simulink model "builtin_block_model_Shunt"  (R2023b)
settings: Solver=VariableStepAuto  StartTime=0.0  StopTime=10  RelTol=1e-3
values from neighbouring files (symbols this model uses):
  J = 0.21    [setup_params_shunt.m]
  LAA = 0.01    [setup_params_shunt.m]
  LFF = 0.167    [setup_params_shunt.m]
  ra = 0.013    [setup_params_shunt.m]
  rf = 1.43    [setup_params_shunt.m]
  Tl = 2.493    [setup_params_shunt.m]
  Va = 24    [setup_params_shunt.m]
libraries: spsControlledVoltageSourceLib x1, spsDCMachineLib x1, sps_lib x1
settings Model: Creator=Noor  LastModifiedBy=USER
settings SolverCC: AlgebraicLoopSolver=TrustRegion
settings DataIOCC: ReturnWorkspaceOutputs=off
settings DebuggingCC: UnconnectedInputMsg=warning  UnconnectedOutputMsg=warning  UnconnectedLineMsg=warning  ArithmeticOperatorsInVariantConditions=warning
settings ModelReferenceCC: EnableRefExpFcnMdlSchedulingChecks=on
settings SFSimCC: SimUseLocalCustomCode=off  CustomCodeUndefinedFunction=UseInterfaceOnly
settings RTWCC: RTWUseLocalCustomCode=off

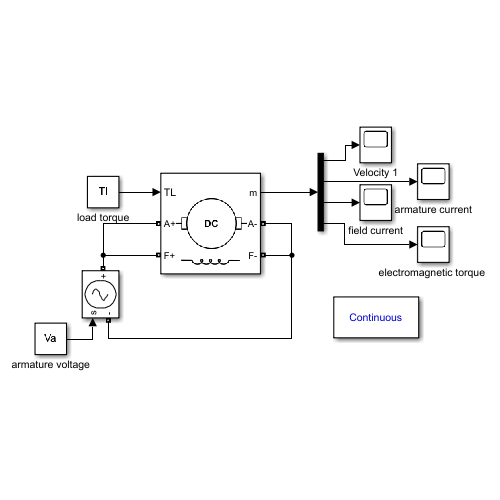
[thumbnail: Simulink's stored preview of the top-level diagram]
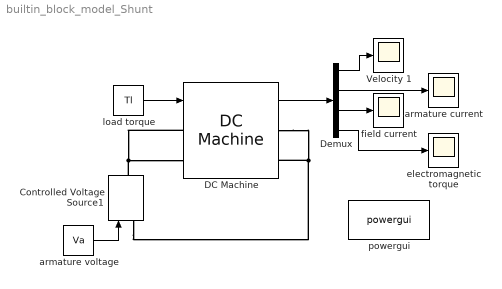
== system builtin_block_model_Shunt ==
  Controlled Voltage Source1 : spsControlledVoltageSourceLib/Controlled Voltage Source  Initialize=on  Source_Type=AC  Amplitude=0  Phase=0  Frequency=0  Measurements=None
  DC Machine : spsDCMachineLib/DC Machine  PresetModel=No  MechanicalLoad=Torque TL  FieldType=Wound  ShowDetailedParameters=on  MeasurementBus=off  RLa=[ra LAA]  RLf=[rf LFF]  Laf=LAF  MachineConstant=Torque constant (N.m/A)  Ke=1.8  Kt=1.8  J=J  Bm=Bm  Tf=0  w0=0  Ifinit=0  TsPowergui=0  TsBlock=-1
  Demux : Demux
  Velocity 1 : Scope
  armature current : Scope
  armature voltage : Constant  Value=Va
  "electromagnetic torque " : Scope
  field current : Scope
  load torque : Constant  Value=Tl
  powergui : sps_lib/powergui  Priority=1  SimulationMode=Continuous  SampleTime=50e-6  frequency=60  Iterations=50  frequencyindice=0  Pbase=100e6  ErrMax=1e-4  UnitsV=kV  UnitsW=MW  buscounter=0  FunctionMessages=off  echomessages=off  EnableUseOfTLC=off  CurrentSourceSwitches=off  DisableSnubberDevices=off  DisableRonSwitches=off  DisableVfSwitches=off  DisplayEquations=off  AutomaticDiscreteSolvers=off  SolverType=Tustin/Backward Euler (TBE)  Interpol=off  ExternalGateDelay=off  methode=off  Ts=100  x0status=blocks  SPID=on  SwTol=0  HookPort=off  NonlinearTolerance=1e-4  nMaxIteration=100  ContinueOnMaxIteration=off  RestoreLinks=warning  ResistiveCurrentMeasurement=off  Frange=[0:2:500]  Ylog=off  Xlog=on  ShowGrid=off  save=off  variable=ZData  structure=0  ZoomFFT=off  StartTime=0.0  cycles=1  DisplayStyle=1  fundamental=60  FreqAxis=off  MaxFrequency=1000  frequencyindicesteady=1  RmsSteady=1  display=off
  wires:
  Demux/3 -> field current/1
  Demux/1 -> Velocity 1/1
  Demux/4 -> "electromagnetic torque "/1
  DC Machine/1 -> Demux/1
  Demux/2 -> armature current/1
  armature voltage/1 -> Controlled Voltage Source1/1
  load torque/1 -> DC Machine/1
  connections:
  Controlled Voltage Source1/RConn1 -- DC Machine/LConn2 -- DC Machine/LConn1
  Controlled Voltage Source1/LConn1 -- DC Machine/RConn2 -- DC Machine/RConn1
